simulink model "WF_offshore"  (R2024a)
settings: Solver=VariableStepAuto  StartTime=0  StopTime=1  RelTol=1e-3
values from neighbouring files (symbols this model uses):
  c_c = 0.177e-6    (= 1.77e-07)    [WF_onshore_SSO_GFL.m]    (also in WF_physical_param_offshore_supersynchronous.m = cable_220(i,6)*1e-9; WF_physical_param_onshore_SSO_020625.m = cable_220(i,6)*1e-9; initialize_params_agg.m)
  c_c_eff = c_c*n_cables    [WF_onshore_SSO_GFL.m]    (also in WF_physical_param_offshore_supersynchronous.m; WF_physical_param_onshore_SSO_020625.m; initialize_params_agg.m)
  cvtr = initialize_NR_VSC_GF(cvtr)    [NR_steadystate_VSC_GF.m]    (also in WF_onshore_SSO_GFL.m = setfield(cvtr,'parameters', p_vary.name,p_vary.val(i)); WF_physical_param_offshore_supersynchronous.m = setfield(cvtr,'parameters', p_vary.name,p_vary.val(i)); WF_physical_param_onshore_SSO_020625.m = setfield(cvtr,'parameters', p_vary.name,p_vary.val(i)); impedance_WT_blackbox.m = base_values(cvtr))
  D_C = 10:4:100    [WF_onshore_SSO_GFL.m]    (also in WF_parameter_variation.m = 10:4:150; WF_physical_param.m = 10:4:150; WF_physical_param_offshore_supersynchronous.m = 50; WF_physical_param_onshore_SSO_020625.m = 50)
  enable_pll = 1    [impedance_WT_agg.m]    (also in initialize_WT_agg.m; initialize_WT_default_gfl.m; initialize_WT_default_offshore_super.m)
  f1 = 50    [WF_onshore_SSO_GFL.m]    (also in WF_physical_param_offshore_supersynchronous.m; WF_physical_param_onshore_SSO_020625.m; initialize_params_agg.m)
  i = 1    [WF_physical_param_offshore_supersynchronous.m]    (also in WF_physical_param_onshore_SSO_020625.m)
  L = inv(R)    [participation_factors_VSC_GF.m]
  l_c = 0.386e-3    (= 0.000386)    [WF_onshore_SSO_GFL.m]    (also in WF_physical_param_offshore_supersynchronous.m = cable_220(i,5)*1e-3; WF_physical_param_onshore_SSO_020625.m = cable_220(i,5)*1e-3; initialize_params_agg.m)
  l_c_eff = l_c/n_cables    [WF_onshore_SSO_GFL.m]    (also in WF_physical_param_offshore_supersynchronous.m; WF_physical_param_onshore_SSO_020625.m; initialize_params_agg.m)
  L_comp = sqrt(2)*l_comp*(Z_b_G/(2*pi*f1))    [WF_physical_param.m]    (also in WF_physical_param_offshore_supersynchronous.m = sqrt(2)*((1/(c_c_eff/2*D_C*2*pi*f1))-(l_tf_wf*(Z_b_G)+(l_c_e; WF_physical_param_onshore_SSO_020625.m = sqrt(2)*((1/(c_c_eff/2*D_C*2*pi*f1))-(l_tf_wf*(Z_b_G)+(l_c_e; initialize_params_agg.m)
  l_OH = 0.2    [WF_onshore_SSO_GFL.m]    (also in WF_physical_param_offshore_supersynchronous.m = 0.1; WF_physical_param_onshore_SSO_020625.m = 0.1; initialize_params_agg.m = 0.1)
  l_tf_wf = tf_params(2,2)    [IM_WF_agg.m]    (also in WF_onshore_SSO_GFL.m = 0.05; WF_physical_param_offshore_supersynchronous.m = 0.05; WF_physical_param_onshore_SSO_020625.m = 0.05; initialize_params_agg.m = 0.05)
  l_tf_wt = tf_params(1,2)    [IM_WF_agg.m]    (also in WF_onshore_SSO_GFL.m = 0.0392; WF_physical_param_offshore_supersynchronous.m = 0.0392; WF_physical_param_onshore_SSO_020625.m = 0.0392; initialize_params_agg.m = 0.0392)
  Lg = p_vary(i)*((Z_b_G/(2*pi*f1)))    [WF_onshore_SSO_GFL.m]    (also in WF_physical_param_offshore_supersynchronous.m; WF_physical_param_onshore_SSO_020625.m; initialize_params_agg.m = 0.1*((Z_b_G/(2*pi*f1))))
  Lg1 = Lg    [WF_physical_param_offshore_supersynchronous.m]    (also in WF_physical_param_onshore_SSO_020625.m)
  Lg2 = Lg    [WF_physical_param_offshore_supersynchronous.m]    (also in WF_physical_param_onshore_SSO_020625.m)
  r_c = 27e-3    (= 0.027)    [WF_onshore_SSO_GFL.m]    (also in WF_physical_param_offshore_supersynchronous.m = cable_220(i,4)*1e-3; WF_physical_param_onshore_SSO_020625.m = cable_220(i,4)*1e-3; initialize_params_agg.m)
  r_c_eff = r_c/n_cables    [WF_onshore_SSO_GFL.m]    (also in WF_physical_param_offshore_supersynchronous.m; WF_physical_param_onshore_SSO_020625.m; initialize_params_agg.m)
  r_diss = .1    (= 0.1)    [WF_physical_param_offshore_supersynchronous.m]    (also in WF_physical_param_onshore_SSO_020625.m; calculate_WF.m; initialize_params_agg.m)
  r_OH = 0.02    [WF_onshore_SSO_GFL.m]    (also in WF_physical_param_offshore_supersynchronous.m = 0.01; WF_physical_param_onshore_SSO_020625.m = 0.01; initialize_params_agg.m)
  r_tf_wf = tf_params(2,1)    [IM_WF_agg.m]    (also in WF_onshore_SSO_GFL.m = 0.005; WF_physical_param_offshore_supersynchronous.m = 0.005; WF_physical_param_onshore_SSO_020625.m = 0.005; initialize_params_agg.m = 0.005)
  r_tf_wt = tf_params(1,1)    [IM_WF_agg.m]    (also in WF_onshore_SSO_GFL.m = 0.0056; WF_physical_param_offshore_supersynchronous.m = 0.0056; WF_physical_param_onshore_SSO_020625.m = 0.0056; initialize_params_agg.m = 0.0056)
  Rg = rg*Z_b_G    [WF_onshore_SSO_GFL.m]    (also in WF_physical_param_offshore_supersynchronous.m; WF_physical_param_onshore_SSO_020625.m; initialize_params_agg.m = 0.01*Z_b_G)
  Sb_WF = (3*1)*5e6    (= 15000000)    [WF_onshore_SSO_GFL.m]    (also in WF_physical_param_offshore_supersynchronous.m; WF_physical_param_onshore_SSO_020625.m; impedance_WT_blackbox.m = n_t*Sb_WT; initialize_params_agg.m = 1000000000)
  Sb_WT = 5e6    (= 5000000)    [IM_WF.m]    (also in WF_onshore_SSO_GFL.m; WF_physical_param_offshore_supersynchronous.m; WF_physical_param_onshore_SSO_020625.m; initialize_params_agg.m)
  selector_current_reference = 3    [impedance_WT_agg.m]    (also in initialize_WT_agg.m; initialize_WT_default_gfl.m; initialize_WT_default_offshore_super.m)
  selector_omega_reference = 1    [impedance_WT_agg.m]    (also in initialize_WT_agg.m; initialize_WT_default_gfl.m; initialize_WT_default_offshore_super.m)
  V_coll = 33e3    (= 33000)    [WF_onshore_SSO_GFL.m]    (also in WF_physical_param_offshore_supersynchronous.m; WF_physical_param_onshore_SSO_020625.m; initialize_params_agg.m)
  V_trans = 220e3    (= 220000)    [WF_onshore_SSO_GFL.m]    (also in WF_physical_param_offshore_supersynchronous.m; WF_physical_param_onshore_SSO_020625.m; initialize_params_agg.m)
  Z_b_G = (V_trans/sqrt(3/2))^2/Sb_WF    [WF_onshore_SSO_GFL.m]    (also in WF_physical_param_offshore_supersynchronous.m = (V_b_trans)^2/Sb_WF; WF_physical_param_onshore_SSO_020625.m = (V_b_trans)^2/Sb_WF; initialize_params_agg.m = (V_b_trans)^2/Sb_WF)
undefined symbols (not defined in the file or in its folder): opts, R
libraries: spsSeriesRLCBranchLib x105, simulink_extras x104, simulink x52, spsThreePhaseVIMeasurementLib x42, spsControlledVoltageSourceLib x42, spsGroundLib x41, spsThreePhaseTransformerTwoWindingsLib x14, powerlib_extras x13, spsVariableInductorLib x9, spsIdealSwitchLib x6, spsVariableCapacitorLib x6, spsThreePhaseSeriesRLCBranchLib x4
(part 7 of 13)

== system WF_offshore/WT_MF8/Inverse Park1 ==
  x_dq : Inport
  delta : Inport  Port=2
  Demux1 : Demux  Outputs=2
  Fcn : Fcn  Expr=cos(u(3))*u(1)-sin(u(3))*u(2)
  Fcn1 : Fcn  Expr=cos(u(3)-2/3*pi)*u(1)-sin(u(3)-2/3*pi)*u(2)
  Fcn2 : Fcn  Expr=cos(u(3)+2/3*pi)*u(1)-sin(u(3)+2/3*pi)*u(2)
  Mux : Mux  Inputs=3
  Mux1 : Mux  Inputs=3
  x_abc : Outport
  wires:
  delta/1 -> Mux/3
  x_dq/1 -> Demux1/1
  Mux1/1 -> x_abc/1
  Fcn2/1 -> Mux1/3
  Fcn1/1 -> Mux1/2
  Fcn/1 -> Mux1/1
  Demux1/1 -> Mux/1
  Demux1/2 -> Mux/2
  Mux/1 -> Fcn/1, Fcn2/1, Fcn1/1

== system WF_offshore/WT_MF8/Subsystem1 ==
  v_abc : Inport
  Controlled Voltage Source : spsControlledVoltageSourceLib/Controlled Voltage Source  Initialize=on  Source_Type=AC  Amplitude=0  Phase=0  Frequency=0  Measurements=None
  Controlled Voltage Source1 : spsControlledVoltageSourceLib/Controlled Voltage Source  Initialize=on  Source_Type=AC  Amplitude=0  Phase=0  Frequency=0  Measurements=None
  Controlled Voltage Source2 : spsControlledVoltageSourceLib/Controlled Voltage Source  Initialize=on  Source_Type=AC  Amplitude=0  Phase=0  Frequency=0  Measurements=None
  Demux : Demux  Outputs=3
  Ground : spsGroundLib/Ground  LConnTagsString=a
  va1 : PMIOPort  Side=Right
  vb1 : PMIOPort  Port=2  Side=Right
  vc1 : PMIOPort  Port=3  Side=Right
  wires:
  Demux/1 -> Controlled Voltage Source/1
  Demux/2 -> Controlled Voltage Source1/1
  Demux/3 -> Controlled Voltage Source2/1
  v_abc/1 -> Demux/1
  connections:
  va1/RConn1 -- Controlled Voltage Source/RConn1
  vb1/RConn1 -- Controlled Voltage Source1/RConn1
  vc1/RConn1 -- Controlled Voltage Source2/RConn1
  Ground/LConn1 -- Controlled Voltage Source2/LConn1 -- Controlled Voltage Source1/LConn1 -- Controlled Voltage Source/LConn1

== system WF_offshore/WT_MF8/Subsystem6 ==
  x_d+ix_q : Inport
  Complex to Real-Imag2 : ComplexToRealImag
  Mux : Mux  Inputs=2
  x_dq : Outport
  wires:
  x_d+ix_q/1 -> Complex to Real-Imag2/1
  Mux/1 -> x_dq/1
  Complex to Real-Imag2/2 -> Mux/2
  Complex to Real-Imag2/1 -> Mux/1

== system WF_offshore/WT_MF8/Transformations (pu and dq) ==
  i_abc_grid : Inport
  i_abc_filt : Inport  Port=2
  v_abc_grid : Inport  Port=3
  v_abc_filt : Inport  Port=4
  Thetavsm : Inport  Port=5
  Thetapll : Inport  Port=6
  3-phase Instantaneous Active & Reactive Power : powerlib_extras/Measurements/3-phase  Instantaneous  Active & Reactive Power
  Demux : Demux  Outputs=2
  Gain : Gain  Gain=1/cvtr.pu.Vb
  Gain1 : Gain  Gain=1/cvtr.pu.Ib
  Gain2 : Gain  Gain=1/cvtr.pu.Sb
  Gain4 : Gain  Gain=1/cvtr.pu.Ib
  Gain6 : Gain  Gain=1/cvtr.pu.Vb
  Park : Subsystem
  Park1 : Subsystem
  Park2 : Subsystem
  Park4 : Subsystem
  Subsystem2 : Subsystem
  Subsystem3 : Subsystem
  Subsystem4 : Subsystem
  Subsystem7 : Subsystem
  io : Outport
  il : Outport  Port=2
  p : Outport  Port=3
  q : Outport  Port=4
  vo_pll : Outport  Port=5
  vo : Outport  Port=6
  wires:
  v_abc_filt/1 -> Gain6/1, Gain/1
  Park2/1(x_dq) -> Subsystem3/1(x_dq)
  Park1/1(x_dq) -> Subsystem4/1(x_dq)
  Park/1(x_dq) -> Subsystem7/1(x_dq)
  Subsystem3/1(x_d+ix_q) -> vo/1
  Subsystem7/1(x_d+ix_q) -> il/1
  Subsystem4/1(x_d+ix_q) -> io/1
  3-phase Instantaneous Active & Reactive Power/1 -> Gain2/1
  v_abc_grid/1 -> 3-phase Instantaneous Active & Reactive Power/1
  Demux/2 -> q/1
  Thetavsm/1 -> Park/2(delta), Park2/2(delta), Park1/2(delta)
  Subsystem2/1(x_d+ix_q) -> vo_pll/1
  Thetapll/1 -> Park4/2(delta)
  i_abc_filt/1 -> Gain4/1
  Demux/1 -> p/1
  Park4/1(x_dq) -> Subsystem2/1(x_dq)
  Gain4/1 -> Park/1(x_abc)
  Gain/1 -> Park2/1(x_abc)
  Gain1/1 -> Park1/1(x_abc)
  Gain2/1 -> Demux/1
  i_abc_grid/1 -> Gain1/1, 3-phase Instantaneous Active & Reactive Power/2
  Gain6/1 -> Park4/1(x_abc)

== system WF_offshore/WT_MF8/filter capacitance1 ==
  Ground : spsGroundLib/Ground  LConnTagsString=a
  Series RLC Branch : spsSeriesRLCBranchLib/Series RLC Branch  LConnTagsString=__new0  RConnTagsString=__new0  BranchType=C  Resistance=R  Inductance=L  SetiL0=on  InitialCurrent=ia0  Capacitance=cvtr.parameters.Cf  Setx0=on  InitialVoltage=cvtr.ss.vo0a  Measurements=None
  Series RLC Branch1 : spsSeriesRLCBranchLib/Series RLC Branch  LConnTagsString=__new0  RConnTagsString=__new0  BranchType=C  Resistance=R  Inductance=L  SetiL0=on  InitialCurrent=ia0  Capacitance=cvtr.parameters.Cf  Setx0=on  InitialVoltage=cvtr.ss.vo0b  Measurements=None
  Series RLC Branch2 : spsSeriesRLCBranchLib/Series RLC Branch  LConnTagsString=__new0  RConnTagsString=__new0  BranchType=C  Resistance=R  Inductance=L  SetiL0=on  InitialCurrent=ia0  Capacitance=cvtr.parameters.Cf  Setx0=on  InitialVoltage=cvtr.ss.vo0c  Measurements=None
  Three-Phase V-I Measurement : spsThreePhaseVIMeasurementLib/Three-Phase V-I Measurement  VoltageMeasurement=phase-to-ground  SetLabelV=off  LabelV=Vabc  Vpu=off  VpuLL=off  CurrentMeasurement=no  SetLabelI=off  LabelI=Iabc  Ipu=off  Pbase=100e6  Vbase=500e3  OutputType=Complex  PhasorSimulation=off  PSBequivalent=0
  A : PMIOPort  Side=Left
  B : PMIOPort  Port=2  Side=Left
  C : PMIOPort  Port=3  Side=Left
  v_abc : Outport
  wires:
  Three-Phase V-I Measurement/1 -> v_abc/1
  connections:
  Series RLC Branch2/RConn1 -- Series RLC Branch1/RConn1 -- Ground/LConn1 -- Series RLC Branch/RConn1
  Three-Phase V-I Measurement/RConn3 -- Series RLC Branch2/LConn1
  Three-Phase V-I Measurement/RConn2 -- Series RLC Branch1/LConn1
  Three-Phase V-I Measurement/RConn1 -- Series RLC Branch/LConn1
  C/RConn1 -- Three-Phase V-I Measurement/LConn3
  B/RConn1 -- Three-Phase V-I Measurement/LConn2
  A/RConn1 -- Three-Phase V-I Measurement/LConn1

== system WF_offshore/WT_MF8/filter inductance1 ==
  Series RLC Branch : spsSeriesRLCBranchLib/Series RLC Branch  LConnTagsString=__new0  RConnTagsString=__new0  BranchType=RL  Resistance=cvtr.parameters.Rf  Inductance=cvtr.parameters.Lf  SetiL0=on  InitialCurrent=cvtr.ss.il0a  Capacitance=1e-6  Setx0=off  InitialVoltage=0  Measurements=None
  Series RLC Branch1 : spsSeriesRLCBranchLib/Series RLC Branch  LConnTagsString=__new0  RConnTagsString=__new0  BranchType=RL  Resistance=cvtr.parameters.Rf  Inductance=cvtr.parameters.Lf  SetiL0=on  InitialCurrent=cvtr.ss.il0b  Capacitance=1e-6  Setx0=off  InitialVoltage=0  Measurements=None
  Series RLC Branch2 : spsSeriesRLCBranchLib/Series RLC Branch  LConnTagsString=__new0  RConnTagsString=__new0  BranchType=RL  Resistance=cvtr.parameters.Rf  Inductance=cvtr.parameters.Lf  SetiL0=on  InitialCurrent=cvtr.ss.il0c  Capacitance=1e-6  Setx0=off  InitialVoltage=0  Measurements=None
  Three-Phase V-I Measurement : spsThreePhaseVIMeasurementLib/Three-Phase V-I Measurement  VoltageMeasurement=no  SetLabelV=off  LabelV=Vabc  Vpu=off  VpuLL=off  CurrentMeasurement=yes  SetLabelI=off  LabelI=Iabc  Ipu=off  Pbase=100e6  Vbase=500e3  OutputType=Complex  PhasorSimulation=off  PSBequivalent=0
  A : PMIOPort  Side=Left
  B : PMIOPort  Port=2  Side=Left
  C : PMIOPort  Port=3  Side=Left
  a : PMIOPort  Port=4  Side=Right
  b : PMIOPort  Port=5  Side=Right
  c : PMIOPort  Port=6  Side=Right
  i_abc : Outport
  wires:
  Three-Phase V-I Measurement/1 -> i_abc/1
  connections:
  Series RLC Branch/RConn1 -- Three-Phase V-I Measurement/LConn1
  Series RLC Branch1/RConn1 -- Three-Phase V-I Measurement/LConn2
  Series RLC Branch2/RConn1 -- Three-Phase V-I Measurement/LConn3
  A/RConn1 -- Series RLC Branch/LConn1
  a/RConn1 -- Three-Phase V-I Measurement/RConn1
  B/RConn1 -- Series RLC Branch1/LConn1
  b/RConn1 -- Three-Phase V-I Measurement/RConn2
  C/RConn1 -- Series RLC Branch2/LConn1
  c/RConn1 -- Three-Phase V-I Measurement/RConn3

== system WF_offshore/WT_MF9/Control System ==
  io : Inport
  il : Inport  Port=2
  p : Inport  Port=3
  q : Inport  Port=4
  vo_pll : Inport  Port=5
  vo : Inport  Port=6
  Add{1..4} (4 alike) : Sum
  Compare To Constant : simulink/Logic and Bit Operations/Compare To Constant  relop===  const=0  OutDataTypeStr=boolean
  Compare To Constant1 : simulink/Logic and Bit Operations/Compare To Constant  relop===  const=1  OutDataTypeStr=boolean
  Compare To Constant2 : simulink/Logic and Bit Operations/Compare To Constant  relop===  const=2  OutDataTypeStr=boolean
  Compare To Constant3 : simulink/Logic and Bit Operations/Compare To Constant  relop===  const=3  OutDataTypeStr=boolean
  Current controller : Subsystem
  Goto2 : Goto  Commented=on  GotoTag=d_pref  TagVisibility=global
  Goto3 : Goto  Commented=on  GotoTag=d_qref  TagVisibility=global
  Goto4 : Goto  Commented=on  GotoTag=d_Oref  TagVisibility=global
  Goto6 : Goto  Commented=on  GotoTag=d_Vref  TagVisibility=global
  Mechanical1 : Subsystem
  Memory : Memory  InitialCondition=cvtr.ss.vir0
  Multiport Switch : MultiPortSwitch  DataPortOrder=Zero-based contiguous  Inputs=4  zeroidx=on  SaturateOnIntegerOverflow=off  InputSameDT=off
  Multiport Switch1 : MultiPortSwitch  DataPortOrder=Zero-based contiguous  Inputs=2  zeroidx=on  SaturateOnIntegerOverflow=off  InputSameDT=off
  Multiport Switch2 : MultiPortSwitch  DataPortOrder=Zero-based contiguous  Inputs=2  zeroidx=on  SaturateOnIntegerOverflow=off  InputSameDT=off
  PLL1 : Subsystem
  PQ controller : Subsystem
  Step : Step  Commented=on  After=0.01  SampleTime=0
  Step1 : Step  Commented=on  Time=1.5  After=0.03  SampleTime=0
  Step2 : Step  Commented=on  Time=2  After=0.001  SampleTime=0
  Step3 : Step  Commented=on  Time=2  After=0.001  SampleTime=0
  Terminator : Terminator
  Terminator1 : Terminator
  Voltage controller DEM : Subsystem
  Voltage controller QSEM : Subsystem
  Voltage controller VCVSM : Subsystem
  delta1 : Constant  Value=cvtr.ss.pref0
  delta2 : Constant  Value=cvtr.ss.DeltaThetavsm0
  delta4 : Constant  Value=cvtr.ss.ilr0
  delta5 : Constant  Value=selector_current_reference
  delta6 : Constant  Value=selector_omega_reference
  io5 : Constant  Value=cvtr.ss.Omegavsm0
  io6 : Constant  Value=cvtr.ss.qref0
  io7 : Constant  Value=cvtr.ss.vref0
  io8 : Constant  Value=cvtr.ss.Omegaref0
  p1 : InportShadow  Port=3
  q droop1 : Subsystem
  q1 : InportShadow  Port=4
  vo3 : InportShadow  Port=6
  vo4 : InportShadow  Port=6
  vo5 : InportShadow  Port=6
  thetapll : Outport
  thetavsm : Outport  Port=2
  vir : Outport  Port=3
  wires:
  io5/1 -> Mechanical1/4(Omegavsm0)
  Voltage controller DEM/1(ilr) -> Multiport Switch/2
  Add1/1 -> [pref], Mechanical1/2(pref)
  delta4/1 -> Voltage controller DEM/4(ilr0)
  Multiport Switch/1 -> Current controller/1(ilr)
  delta2/1 -> Mechanical1/3(DeltaThetavsm0)
  Add2/1 -> [qref], q droop1/2(qref)  "qref"
  delta1/1 -> Add1/2  "pref"
  q droop1/2(qm) -> Terminator/1  "qm"
  Add4/1 -> Mechanical1/5(Omegaref)  "omegaref"
  io7/1 -> Add3/2  "vref0"
  [Omegavsm] -> Voltage controller QSEM/3(Omegavsm)
  io8/1 -> Add4/2  "omegaref0"
  Step/1 -> Add1/1, Goto2/1  "dPref"
  [ve] -> Voltage controller QSEM/1(ve)
  delta5/1 -> Compare To Constant3/1, Compare To Constant2/1, Compare To Constant1/1, Multiport Switch/1, Compare To Constant/1
  io6/1 -> Add2/2  "qref0"
  Add3/1 -> q droop1/3(vref)  "vref"
  q/1 -> q droop1/1(q)
  [Omegavsm] -> Voltage controller VCVSM/2(Omega)
  [ve] -> Voltage controller DEM/1(ve)
  [Omegapll] -> Mechanical1/6(Omegapll)
  [Omegavsm] -> Voltage controller DEM/3(Omegavsm)
  p/1 -> Mechanical1/1(p)
  Voltage controller VCVSM/1(ilr) -> Multiport Switch/4
  vo/1 -> Voltage controller QSEM/2(vo)
  vo_pll/1 -> PLL1/1(vo)
  PLL1/2(vpll) -> Terminator1/1  "vpll"
  q droop1/1(ve) -> [ve]
  Voltage controller QSEM/1(ilr) -> Multiport Switch/3
  Memory/1 -> vir/1
  Current controller/1(vir) -> Memory/1
  p1/1 -> PQ controller/2(p)
  q1/1 -> PQ controller/4(q)
  PQ controller/1(ir) -> Multiport Switch/5
  il/1 -> Current controller/2(il)
  delta6/1 -> Multiport Switch2/1, Multiport Switch1/1
  [Omegapll] -> Current controller/3(Omega)
  Mechanical1/2(Omegavsm) -> Multiport Switch1/2  "wvsm"
  [Omegapll] -> Multiport Switch1/3
  Multiport Switch2/1 -> thetavsm/1
  Mechanical1/1(Thetavsm) -> Multiport Switch2/2  "thetavsm"
  Compare To Constant/1 -> Voltage controller DEM/Enable
  Compare To Constant1/1 -> Voltage controller QSEM/Enable
  Compare To Constant2/1 -> Voltage controller VCVSM/Enable
  Compare To Constant3/1 -> PQ controller/Enable
  Multiport Switch1/1 -> [Omegavsm]
  PLL1/1(Omegapll) -> [Omegapll]
  PLL1/3(Thetapll) -> Multiport Switch2/3, thetapll/1  "thetapll"
  io/1 -> Voltage controller VCVSM/3(io)
  vo3/1 -> Current controller/4(vo)
  vo4/1 -> Voltage controller DEM/2(vo)
  vo5/1 -> Voltage controller VCVSM/1(vo)
  [ve] -> Voltage controller VCVSM/4(ve)
  [pref] -> PQ controller/1(pref)
  [qref] -> PQ controller/3(qref)
  Step1/1 -> Goto3/1, Add2/1  "dQref"
  Step2/1 -> Add4/1, Goto4/1  "dOmegaref"
  Step3/1 -> Add3/1, Goto6/1  "dVref"

== system WF_offshore/WT_MF9/Inverse Park1 ==
  x_dq : Inport
  delta : Inport  Port=2
  Demux1 : Demux  Outputs=2
  Fcn : Fcn  Expr=cos(u(3))*u(1)-sin(u(3))*u(2)
  Fcn1 : Fcn  Expr=cos(u(3)-2/3*pi)*u(1)-sin(u(3)-2/3*pi)*u(2)
  Fcn2 : Fcn  Expr=cos(u(3)+2/3*pi)*u(1)-sin(u(3)+2/3*pi)*u(2)
  Mux : Mux  Inputs=3
  Mux1 : Mux  Inputs=3
  x_abc : Outport
  wires:
  Mux/1 -> Fcn1/1, Fcn2/1, Fcn/1
  Demux1/2 -> Mux/2
  Demux1/1 -> Mux/1
  Fcn/1 -> Mux1/1
  Fcn1/1 -> Mux1/2
  Fcn2/1 -> Mux1/3
  Mux1/1 -> x_abc/1
  x_dq/1 -> Demux1/1
  delta/1 -> Mux/3

== system WF_offshore/WT_MF9/Subsystem1 ==
  v_abc : Inport
  Controlled Voltage Source : spsControlledVoltageSourceLib/Controlled Voltage Source  Initialize=on  Source_Type=AC  Amplitude=0  Phase=0  Frequency=0  Measurements=None
  Controlled Voltage Source1 : spsControlledVoltageSourceLib/Controlled Voltage Source  Initialize=on  Source_Type=AC  Amplitude=0  Phase=0  Frequency=0  Measurements=None
  Controlled Voltage Source2 : spsControlledVoltageSourceLib/Controlled Voltage Source  Initialize=on  Source_Type=AC  Amplitude=0  Phase=0  Frequency=0  Measurements=None
  Demux : Demux  Outputs=3
  Ground : spsGroundLib/Ground  LConnTagsString=a
  va1 : PMIOPort  Side=Right
  vb1 : PMIOPort  Port=2  Side=Right
  vc1 : PMIOPort  Port=3  Side=Right
  wires:
  v_abc/1 -> Demux/1
  Demux/3 -> Controlled Voltage Source2/1
  Demux/2 -> Controlled Voltage Source1/1
  Demux/1 -> Controlled Voltage Source/1
  connections:
  Controlled Voltage Source/LConn1 -- Controlled Voltage Source1/LConn1 -- Controlled Voltage Source2/LConn1 -- Ground/LConn1
  vc1/RConn1 -- Controlled Voltage Source2/RConn1
  vb1/RConn1 -- Controlled Voltage Source1/RConn1
  va1/RConn1 -- Controlled Voltage Source/RConn1

== system WF_offshore/WT_MF9/Subsystem6 ==
  x_d+ix_q : Inport
  Complex to Real-Imag2 : ComplexToRealImag
  Mux : Mux  Inputs=2
  x_dq : Outport
  wires:
  Complex to Real-Imag2/1 -> Mux/1
  Complex to Real-Imag2/2 -> Mux/2
  Mux/1 -> x_dq/1
  x_d+ix_q/1 -> Complex to Real-Imag2/1

== system WF_offshore/WT_MF9/Transformations (pu and dq) ==
  i_abc_grid : Inport
  i_abc_filt : Inport  Port=2
  v_abc_grid : Inport  Port=3
  v_abc_filt : Inport  Port=4
  Thetavsm : Inport  Port=5
  Thetapll : Inport  Port=6
  3-phase Instantaneous Active & Reactive Power : powerlib_extras/Measurements/3-phase  Instantaneous  Active & Reactive Power
  Demux : Demux  Outputs=2
  Gain : Gain  Gain=1/cvtr.pu.Vb
  Gain1 : Gain  Gain=1/cvtr.pu.Ib
  Gain2 : Gain  Gain=1/cvtr.pu.Sb
  Gain4 : Gain  Gain=1/cvtr.pu.Ib
  Gain6 : Gain  Gain=1/cvtr.pu.Vb
  Park : Subsystem
  Park1 : Subsystem
  Park2 : Subsystem
  Park4 : Subsystem
  Subsystem2 : Subsystem
  Subsystem3 : Subsystem
  Subsystem4 : Subsystem
  Subsystem7 : Subsystem
  io : Outport
  il : Outport  Port=2
  p : Outport  Port=3
  q : Outport  Port=4
  vo_pll : Outport  Port=5
  vo : Outport  Port=6
  wires:
  Gain6/1 -> Park4/1(x_abc)
  i_abc_grid/1 -> 3-phase Instantaneous Active & Reactive Power/2, Gain1/1
  Gain2/1 -> Demux/1
  Gain1/1 -> Park1/1(x_abc)
  Gain/1 -> Park2/1(x_abc)
  Gain4/1 -> Park/1(x_abc)
  Park4/1(x_dq) -> Subsystem2/1(x_dq)
  Demux/1 -> p/1
  i_abc_filt/1 -> Gain4/1
  Thetapll/1 -> Park4/2(delta)
  Subsystem2/1(x_d+ix_q) -> vo_pll/1
  Thetavsm/1 -> Park1/2(delta), Park2/2(delta), Park/2(delta)
  Demux/2 -> q/1
  v_abc_grid/1 -> 3-phase Instantaneous Active & Reactive Power/1
  3-phase Instantaneous Active & Reactive Power/1 -> Gain2/1
  Subsystem4/1(x_d+ix_q) -> io/1
  Subsystem7/1(x_d+ix_q) -> il/1
  Subsystem3/1(x_d+ix_q) -> vo/1
  Park/1(x_dq) -> Subsystem7/1(x_dq)
  Park1/1(x_dq) -> Subsystem4/1(x_dq)
  Park2/1(x_dq) -> Subsystem3/1(x_dq)
  v_abc_filt/1 -> Gain/1, Gain6/1

== system WF_offshore/WT_MF9/filter capacitance1 ==
  Ground : spsGroundLib/Ground  LConnTagsString=a
  Series RLC Branch : spsSeriesRLCBranchLib/Series RLC Branch  LConnTagsString=__new0  RConnTagsString=__new0  BranchType=C  Resistance=R  Inductance=L  SetiL0=on  InitialCurrent=ia0  Capacitance=cvtr.parameters.Cf  Setx0=on  InitialVoltage=cvtr.ss.vo0a  Measurements=None
  Series RLC Branch1 : spsSeriesRLCBranchLib/Series RLC Branch  LConnTagsString=__new0  RConnTagsString=__new0  BranchType=C  Resistance=R  Inductance=L  SetiL0=on  InitialCurrent=ia0  Capacitance=cvtr.parameters.Cf  Setx0=on  InitialVoltage=cvtr.ss.vo0b  Measurements=None
  Series RLC Branch2 : spsSeriesRLCBranchLib/Series RLC Branch  LConnTagsString=__new0  RConnTagsString=__new0  BranchType=C  Resistance=R  Inductance=L  SetiL0=on  InitialCurrent=ia0  Capacitance=cvtr.parameters.Cf  Setx0=on  InitialVoltage=cvtr.ss.vo0c  Measurements=None
  Three-Phase V-I Measurement : spsThreePhaseVIMeasurementLib/Three-Phase V-I Measurement  VoltageMeasurement=phase-to-ground  SetLabelV=off  LabelV=Vabc  Vpu=off  VpuLL=off  CurrentMeasurement=no  SetLabelI=off  LabelI=Iabc  Ipu=off  Pbase=100e6  Vbase=500e3  OutputType=Complex  PhasorSimulation=off  PSBequivalent=0
  A : PMIOPort  Side=Left
  B : PMIOPort  Port=2  Side=Left
  C : PMIOPort  Port=3  Side=Left
  v_abc : Outport
  wires:
  Three-Phase V-I Measurement/1 -> v_abc/1
  connections:
  A/RConn1 -- Three-Phase V-I Measurement/LConn1
  B/RConn1 -- Three-Phase V-I Measurement/LConn2
  C/RConn1 -- Three-Phase V-I Measurement/LConn3
  Three-Phase V-I Measurement/RConn1 -- Series RLC Branch/LConn1
  Three-Phase V-I Measurement/RConn2 -- Series RLC Branch1/LConn1
  Three-Phase V-I Measurement/RConn3 -- Series RLC Branch2/LConn1
  Series RLC Branch/RConn1 -- Ground/LConn1 -- Series RLC Branch1/RConn1 -- Series RLC Branch2/RConn1

== system WF_offshore/WT_MF9/filter inductance1 ==
  Series RLC Branch : spsSeriesRLCBranchLib/Series RLC Branch  LConnTagsString=__new0  RConnTagsString=__new0  BranchType=RL  Resistance=cvtr.parameters.Rf  Inductance=cvtr.parameters.Lf  SetiL0=on  InitialCurrent=cvtr.ss.il0a  Capacitance=1e-6  Setx0=off  InitialVoltage=0  Measurements=None
  Series RLC Branch1 : spsSeriesRLCBranchLib/Series RLC Branch  LConnTagsString=__new0  RConnTagsString=__new0  BranchType=RL  Resistance=cvtr.parameters.Rf  Inductance=cvtr.parameters.Lf  SetiL0=on  InitialCurrent=cvtr.ss.il0b  Capacitance=1e-6  Setx0=off  InitialVoltage=0  Measurements=None
  Series RLC Branch2 : spsSeriesRLCBranchLib/Series RLC Branch  LConnTagsString=__new0  RConnTagsString=__new0  BranchType=RL  Resistance=cvtr.parameters.Rf  Inductance=cvtr.parameters.Lf  SetiL0=on  InitialCurrent=cvtr.ss.il0c  Capacitance=1e-6  Setx0=off  InitialVoltage=0  Measurements=None
  Three-Phase V-I Measurement : spsThreePhaseVIMeasurementLib/Three-Phase V-I Measurement  VoltageMeasurement=no  SetLabelV=off  LabelV=Vabc  Vpu=off  VpuLL=off  CurrentMeasurement=yes  SetLabelI=off  LabelI=Iabc  Ipu=off  Pbase=100e6  Vbase=500e3  OutputType=Complex  PhasorSimulation=off  PSBequivalent=0
  A : PMIOPort  Side=Left
  B : PMIOPort  Port=2  Side=Left
  C : PMIOPort  Port=3  Side=Left
  a : PMIOPort  Port=4  Side=Right
  b : PMIOPort  Port=5  Side=Right
  c : PMIOPort  Port=6  Side=Right
  i_abc : Outport
  wires:
  Three-Phase V-I Measurement/1 -> i_abc/1
  connections:
  c/RConn1 -- Three-Phase V-I Measurement/RConn3
  C/RConn1 -- Series RLC Branch2/LConn1
  b/RConn1 -- Three-Phase V-I Measurement/RConn2
  B/RConn1 -- Series RLC Branch1/LConn1
  a/RConn1 -- Three-Phase V-I Measurement/RConn1
  A/RConn1 -- Series RLC Branch/LConn1
  Series RLC Branch2/RConn1 -- Three-Phase V-I Measurement/LConn3
  Series RLC Branch1/RConn1 -- Three-Phase V-I Measurement/LConn2
  Series RLC Branch/RConn1 -- Three-Phase V-I Measurement/LConn1

== system WF_offshore/WT_MF1/Control System/Current controller ==
  note: Active damping
  note: Feedforward
  note: Decoupling term
  note: PI regulator
  ilr : Inport
  il : Inport  Port=2
  Omega : Inport  Port=3
  vo : Inport  Port=4
  Gain : Gain  Gain=cvtr.parameters.kpc
  Gain1 : Gain
  Gain2 : Gain  Gain=cvtr.parameters.kic
  Gain3 : Gain  Gain=1i*cvtr.parameters.lf
  Gain4 : Gain  Gain=cvtr.parameters.kffv
  Gain5 : Gain  Gain=cvtr.parameters.kad
  Product : Product  RndMeth=Zero
  Subsystem : Subsystem
  Subsystem1 : Subsystem  mask{Omega=cvtr.parameters.Omegaad, xd0=cvtr.ss.Phid0, xq0=cvtr.ss.Phiq0}
  Subtract1 : Sum  Inputs=|++
  Subtract2 : Sum  Inputs=|++
  Subtract3 : Sum  Inputs=|+-
  Subtract4 : Sum  Inputs=|+-
  Subtract5 : Sum  Inputs=|++
  Subtract6 : Sum  Inputs=|+-
  delta1 : Constant  Value=cvtr.ss.Gamma0
  il1 : InportShadow  Port=2
  vo1 : InportShadow  Port=4
  vir : Outport
  wires:
  Gain2/1 -> Subtract1/2
  Gain3/1 -> Subtract2/2
  Product/1 -> Gain3/1
  Omega/1 -> Product/2
  vo/1 -> Gain4/1
  Gain4/1 -> Subtract5/2
  Gain5/1 -> Subtract6/2
  Subtract4/1 -> Gain5/1
  delta1/1 -> Subsystem/2(x0)
  il/1 -> Subtract3/2
  Subsystem/1(x/s) -> Gain2/1  "Gamma"
  il1/1 -> Product/1
  Subtract1/1 -> Subtract2/1
  vo1/1 -> Subsystem1/1(in), Subtract4/1
  Subsystem1/1(out) -> Subtract4/2
  Subtract2/1 -> Subtract5/1
  Subtract5/1 -> Subtract6/1
  Gain/1 -> Subtract1/1
  Subtract6/1 -> Gain1/1
  Gain1/1 -> vir/1
  Subtract3/1 -> Subsystem/1(x), Gain/1
  ilr/1 -> Subtract3/1

== system WF_offshore/WT_MF1/Control System/Mechanical1 ==
  p : Inport
  pref : Inport  Port=2
  DeltaThetavsm0 : Inport  Port=3
  Omegavsm0 : Inport  Port=4
  Omegaref : Inport  Port=5
  Omegapll : Inport  Port=6
  Constant : Constant  Value=enable_pll
  Gain : Gain  Gain=1/cvtr.parameters.ta
  Gain1 : Gain  Gain=cvtr.parameters.kd
  Gain2 : Gain  Gain=cvtr.parameters.kdrpOmega
  Gain3 : Gain  Gain=cvtr.pu.Omegab
  Integrator1 : Integrator  InitialConditionSource=external
  Integrator2 : Integrator  InitialConditionSource=external
  Subtract : Sum  Inputs=-+--
  Subtract1 : Sum  Inputs=-+
  Subtract2 : Sum  Inputs=-+
  Switch : Switch  Criteria=u2 > Threshold  SaturateOnIntegerOverflow=off  InputSameDT=off
  Transfer Fcn (with initial outputs) : simulink_extras/Additional Linear/Transfer Fcn (with initial outputs)  N=[cvtr.parameters.Omegadf]  D="[1  cvtr.parameters.Omegadf]"  Y0=cvtr.ss.Kappa0  U0=cvtr.ss.Kappa0
  Thetavsm : Outport
  Omegavsm : Outport  Port=2
  wires:
  DeltaThetavsm0/1 -> Integrator1/2
  p/1 -> Subtract/1
  pref/1 -> Subtract/2
  Subtract/1 -> Gain/1
  Gain1/1 -> Subtract/3
  Subtract1/1 -> Gain1/1
  Omegavsm0/1 -> Integrator2/2
  Gain/1 -> Integrator2/1
  Omegaref/1 -> Subtract2/1
  Subtract2/1 -> Gain2/1
  Gain2/1 -> Subtract/4
  Gain3/1 -> Integrator1/1
  Omegapll/1 -> Switch/1
  Constant/1 -> Switch/2
  Transfer Fcn (with initial outputs)/1 -> Switch/3
  Integrator2/1 -> Gain3/1, Transfer Fcn (with initial outputs)/1, Subtract2/2, Subtract1/2, Omegavsm/1
  Switch/1 -> Subtract1/1
  Integrator1/1 -> Thetavsm/1

== system WF_offshore/WT_MF1/Control System/PLL1 ==
  note: DeltaOmegapll
  vo : Inport
  Add : Sum
  Add3 : Sum
  Constant : Constant  Value=cvtr.ss.Epsilonpll0
  Constant1 : Constant  Value=cvtr.ss.DeltaThetapll0
  Constant3 : Constant  Value=-cvtr.ss.DeltaThetapll0
  Constant4 : Constant  Value=cvtr.parameters.Omegan
  Demux : Demux  Outputs=2
  Demux1 : Demux  Outputs=2
  Gain : Gain  Gain=cvtr.parameters.kppll
  Gain1 : Gain  Gain=cvtr.pu.Omegab
  Gain2 : Gain  Gain=cvtr.parameters.kipll
  Integrator1 : Integrator  InitialConditionSource=external
  Integrator2 : Integrator  InitialConditionSource=external
  Multiport Switch1 : MultiPortSwitch  DataPortOrder=Zero-based contiguous  Inputs=2  zeroidx=on  SaturateOnIntegerOverflow=off  InputSameDT=off
  Mux : Mux  Inputs=2
  Subsystem1 : Subsystem
  Subsystem3 : Subsystem
  Terminator : Terminator
  Terminator1 : Terminator
  Transfer Fcn (with initial outputs) : simulink_extras/Additional Linear/Transfer Fcn (with initial outputs)  N=[cvtr.parameters.Omegalppll]  D="[1  cvtr.parameters.Omegalppll]"  Y0=real(cvtr.ss.vpll0)  U0=real(cvtr.ss.vpll0)
  Transfer Fcn (with initial outputs)1 : simulink_extras/Additional Linear/Transfer Fcn (with initial outputs)  N=[cvtr.parameters.Omegalppll]  D="[1  cvtr.parameters.Omegalppll]"  Y0=imag(cvtr.ss.vpll0)  U0=imag(cvtr.ss.vpll0)
  Trigonometric Function : Trigonometry  Operator=atan2
  delta6 : Constant  Value=selector_omega_reference
  Omegapll : Outport
  vpll : Outport  Port=2
  Thetapll : Outport  Port=3
  wires:
  vo/1 -> Subsystem1/1(x_d+ix_q)
  Subsystem1/1(x_dq) -> Demux/1
  Transfer Fcn (with initial outputs)1/1 -> Trigonometric Function/1, Mux/2
  Trigonometric Function/1 -> Integrator2/1, Gain/1
  Gain/1 -> Add/1
  Constant/1 -> Integrator2/2
  Gain2/1 -> Add/2
  Add/1 -> Add3/2
  Subsystem3/1(x_d+ix_q) -> vpll/1
  Add3/1 -> Omegapll/1, Gain1/1
  Constant4/1 -> Add3/1
  Gain1/1 -> Integrator1/1
  Mux/1 -> Demux1/1, Subsystem3/1(x_dq)
  Demux1/2 -> Terminator1/1  "vpll_q"
  Demux1/1 -> Terminator/1  "vpll_d"
  Demux/1 -> Transfer Fcn (with initial outputs)/1
  Transfer Fcn (with initial outputs)/1 -> Mux/1, Trigonometric Function/2
  Integrator2/1 -> Gain2/1
  Integrator1/1 -> Thetapll/1
  Constant3/1 -> Multiport Switch1/3
  delta6/1 -> Multiport Switch1/1
  Constant1/1 -> Multiport Switch1/2
  Multiport Switch1/1 -> Integrator1/2
  Demux/2 -> Transfer Fcn (with initial outputs)1/1

== system WF_offshore/WT_MF1/Control System/PQ controller ==
  note: PI regulator
  note: PI regulator
  pref : Inport
  p : Inport  Port=2
  qref : Inport  Port=3
  q : Inport  Port=4
  Enable : EnablePort
  Gain : Gain  Gain=cvtr.parameters.kpp
  Gain1 : Gain  Gain=cvtr.parameters.kpq
  Gain2 : Gain  Gain=cvtr.parameters.kip
  Gain3 : Gain  Gain=cvtr.parameters.kiq
  Gain4 : Gain
  Gain5 : Gain  Gain=-1
  Integrator1 : Integrator  InitialConditionSource=external
  Integrator2 : Integrator  InitialConditionSource=external
  Mux : Mux  Inputs=2
  Subsystem3 : Subsystem
  Subtract1 : Sum  Inputs=|++
  Subtract2 : Sum  Inputs=|++
  Subtract3 : Sum  Inputs=|+-
  Subtract4 : Sum  Inputs=|+-
  delta1 : Constant  Value=cvtr.ss.GammaSd0
  delta2 : Constant  Value=cvtr.ss.GammaSq0
  ir : Outport
  wires:
  Gain/1 -> Subtract1/1
  Integrator1/1 -> Gain2/1
  p/1 -> Subtract3/2
  Subtract3/1 -> Integrator1/1, Gain/1
  delta1/1 -> Integrator1/2
  Gain2/1 -> Subtract1/2
  pref/1 -> Subtract3/1
  qref/1 -> Subtract4/1
  Gain3/1 -> Subtract2/2
  delta2/1 -> Integrator2/2
  Subtract4/1 -> Integrator2/1, Gain1/1
  q/1 -> Subtract4/2
  Integrator2/1 -> Gain3/1
  Gain1/1 -> Subtract2/1
  Mux/1 -> Subsystem3/1(x_dq)
  Subtract1/1 -> Gain4/1
  Subtract2/1 -> Gain5/1
  Subsystem3/1(x_d+ix_q) -> ir/1
  Gain5/1 -> Mux/2
  Gain4/1 -> Mux/1

== system WF_offshore/WT_MF1/Control System/Voltage controller DEM ==
  ve : Inport
  vo : Inport  Port=2
  Omegavsm : Inport  Port=3
  ilr0 : Inport  Port=4
  Enable : EnablePort
  Gain : Gain  Gain=cvtr.pu.Omegab/cvtr.parameters.ls
  Gain1 : Gain  Gain=cvtr.pu.Omegab/cvtr.parameters.ls
  Gain2 : Gain  Gain=cvtr.pu.Omegab*cvtr.parameters.rs/cvtr.parameters.ls
  Gain3 : Gain  Gain=1i*cvtr.pu.Omegab
  Product : Product  RndMeth=Zero
  Subsystem : Subsystem
  Subtract : Sum  Inputs=+---
  ilr : Outport
  wires:
  Omegavsm/1 -> Product/2
  Product/1 -> Gain3/1
  Gain3/1 -> Subtract/4
  Gain2/1 -> Subtract/3
  Subtract/1 -> Subsystem/1(x)
  Gain1/1 -> Subtract/2
  vo/1 -> Gain1/1
  Gain/1 -> Subtract/1
  ve/1 -> Gain/1
  Subsystem/1(x/s) -> Product/1, Gain2/1, ilr/1
  ilr0/1 -> Subsystem/2(x0)

== system WF_offshore/WT_MF1/Control System/Voltage controller QSEM ==
  ve : Inport
  vo : Inport  Port=2
  Omegavsm : Inport  Port=3
  Enable : EnablePort
  Constant : Constant  Value=cvtr.pu.Omegab*cvtr.parameters.rs/cvtr.parameters.ls
  Demux : Demux  Outputs=2
  Demux1 : Demux  Outputs=2
  Divide : Product  Inputs=*/
  Gain : Gain  Gain=cvtr.pu.Omegab/cvtr.parameters.ls
  Gain1 : Gain  Gain=cvtr.pu.Omegab/cvtr.parameters.ls
  Gain3 : Gain  Gain=1i*cvtr.pu.Omegab
  Mux : Mux  Inputs=2
  Subsystem2 : Subsystem
  Subsystem3 : Subsystem
  Subtract : Sum  Inputs=+-
  Subtract1 : Sum
  Terminator : Terminator
  Terminator1 : Terminator
  Transfer Fcn (with initial outputs) : simulink_extras/Additional Linear/Transfer Fcn (with initial outputs)  N=[cvtr.parameters.Omegavo]  D="[1  cvtr.parameters.Omegavo]"  Y0=cvtr.ss.vomd0  U0=cvtr.ss.vomd0
  Transfer Fcn (with initial outputs)1 : simulink_extras/Additional Linear/Transfer Fcn (with initial outputs)  N=[cvtr.parameters.Omegavo]  D="[1  cvtr.parameters.Omegavo]"  Y0=cvtr.ss.vomq0  U0=cvtr.ss.vomq0
  ilr : Outport
  wires:
  Omegavsm/1 -> Gain3/1
  Gain3/1 -> Subtract1/2
  Gain1/1 -> Subtract/2
  Gain/1 -> Subtract/1
  ve/1 -> Gain/1
  Subtract/1 -> Divide/1
  Constant/1 -> Subtract1/1
  Divide/1 -> ilr/1
  Subtract1/1 -> Divide/2
  vo/1 -> Subsystem2/1(x_d+ix_q)
  Subsystem2/1(x_dq) -> Demux/1
  Transfer Fcn (with initial outputs)/1 -> Mux/1
  Mux/1 -> Demux1/1, Subsystem3/1(x_dq)
  Subsystem3/1(x_d+ix_q) -> Gain1/1
  Demux1/1 -> Terminator/1  "vomd?"
  Demux1/2 -> Terminator1/1  "vomq?"
  Demux/1 -> Transfer Fcn (with initial outputs)/1
  Demux/2 -> Transfer Fcn (with initial outputs)1/1
  Transfer Fcn (with initial outputs)1/1 -> Mux/2

== system WF_offshore/WT_MF1/Control System/Voltage controller VCVSM ==
  note: Voltage controller
  note: Feedforward
  note: Decoupling term
  note: PI regulator
  vo : Inport
  Omega : Inport  Port=2
  io : Inport  Port=3
  ve : Inport  Port=4
  Enable : EnablePort
  Gain : Gain  Gain=cvtr.parameters.kpv
  Gain1 : Gain  Gain=cvtr.parameters.rs
  Gain2 : Gain  Gain=cvtr.parameters.kiv
  Gain3 : Gain  Gain=1i*cvtr.parameters.cf
  Gain4 : Gain  Gain=cvtr.parameters.kffi
  Gain5 : Gain  Gain=1i*cvtr.parameters.ls
  Omega1 : InportShadow  Port=2
  Product : Product  RndMeth=Zero
  Product1 : Product
  Subsystem : Subsystem
  Subtract : Sum  Inputs=+--
  Subtract1 : Sum  Inputs=|++
  Subtract2 : Sum  Inputs=|++
  Subtract3 : Sum  Inputs=|+-
  Subtract5 : Sum  Inputs=|++
  delta1 : Constant  Value=cvtr.ss.Xi0
  io1 : InportShadow  Port=3
  vo1 : InportShadow
  ilr : Outport
  wires:
  Subtract/1 -> Subtract3/1  "vor"
  Gain/1 -> Subtract1/1
  Gain2/1 -> Subtract1/2
  Gain3/1 -> Subtract2/2
  Product/1 -> Gain3/1
  Omega/1 -> Product/2
  io/1 -> Gain4/1
  Gain4/1 -> Subtract5/2
  delta1/1 -> Subsystem/2(x0)
  Subtract3/1 -> Gain/1, Subsystem/1(x)
  vo/1 -> Subtract3/2
  Subsystem/1(x/s) -> Gain2/1  "Xi"
  vo1/1 -> Product/1
  Subtract1/1 -> Subtract2/1
  Subtract2/1 -> Subtract5/1
  Subtract5/1 -> ilr/1
  io1/1 -> Gain1/1, Product1/1
  Omega1/1 -> Product1/2
  Gain5/1 -> Subtract/3
  Product1/1 -> Gain5/1
  ve/1 -> Subtract/1
  Gain1/1 -> Subtract/2

== system WF_offshore/WT_MF1/Control System/q droop1 ==
  q : Inport
  qref : Inport  Port=2
  vref : Inport  Port=3
  Gain3 : Gain  Gain=cvtr.parameters.kdrpq
  Subtract : Sum
  Subtract3 : Sum  Inputs=-+
  Transfer Fcn (with initial outputs) : simulink_extras/Additional Linear/Transfer Fcn (with initial outputs)  N=[cvtr.parameters.Omegaqf]  D="[1  cvtr.parameters.Omegaqf]"  Y0=cvtr.ss.q0  U0=cvtr.ss.q0
  ve : Outport
  qm : Outport  Port=2
  wires:
  vref/1 -> Subtract/2
  qref/1 -> Subtract3/2
  Transfer Fcn (with initial outputs)/1 -> Subtract3/1, qm/1
  Subtract3/1 -> Gain3/1
  Gain3/1 -> Subtract/1
  Subtract/1 -> ve/1
  q/1 -> Transfer Fcn (with initial outputs)/1

== system WF_offshore/WT_MF1/Transformations (pu and dq)/Park ==
  x_abc : Inport
  delta : Inport  Port=2
  Demux1 : Demux  Outputs=3
  Fcn : Fcn  Expr=2/3*(cos(u(4))*u(1)+cos(u(4)-2/3*pi)*u(2)+cos(u(4)+2/3*pi)*u(3))
  Fcn1 : Fcn  Expr=-2/3*(sin(u(4))*u(1)+sin(u(4)-2/3*pi)*u(2)+sin(u(4)+2/3*pi)*u(3))
  Mux : Mux
  Mux1 : Mux  Inputs=2
  x_dq : Outport
  wires:
  Demux1/1 -> Mux/1
  Demux1/2 -> Mux/2
  Demux1/3 -> Mux/3
  x_abc/1 -> Demux1/1
  delta/1 -> Mux/4
  Mux/1 -> Fcn/1, Fcn1/1
  Fcn/1 -> Mux1/1
  Fcn1/1 -> Mux1/2
  Mux1/1 -> x_dq/1

== system WF_offshore/WT_MF1/Transformations (pu and dq)/Park1 ==
  x_abc : Inport
  delta : Inport  Port=2
  Demux1 : Demux  Outputs=3
  Fcn : Fcn  Expr=2/3*(cos(u(4))*u(1)+cos(u(4)-2/3*pi)*u(2)+cos(u(4)+2/3*pi)*u(3))
  Fcn1 : Fcn  Expr=-2/3*(sin(u(4))*u(1)+sin(u(4)-2/3*pi)*u(2)+sin(u(4)+2/3*pi)*u(3))
  Mux : Mux
  Mux1 : Mux  Inputs=2
  x_dq : Outport
  wires:
  Mux1/1 -> x_dq/1
  Fcn1/1 -> Mux1/2
  Fcn/1 -> Mux1/1
  Mux/1 -> Fcn1/1, Fcn/1
  delta/1 -> Mux/4
  x_abc/1 -> Demux1/1
  Demux1/3 -> Mux/3
  Demux1/2 -> Mux/2
  Demux1/1 -> Mux/1

== system WF_offshore/WT_MF1/Transformations (pu and dq)/Park2 ==
  x_abc : Inport
  delta : Inport  Port=2
  Demux1 : Demux  Outputs=3
  Fcn : Fcn  Expr=2/3*(cos(u(4))*u(1)+cos(u(4)-2/3*pi)*u(2)+cos(u(4)+2/3*pi)*u(3))
  Fcn1 : Fcn  Expr=-2/3*(sin(u(4))*u(1)+sin(u(4)-2/3*pi)*u(2)+sin(u(4)+2/3*pi)*u(3))
  Mux : Mux
  Mux1 : Mux  Inputs=2
  x_dq : Outport
  wires:
  Mux1/1 -> x_dq/1
  Fcn1/1 -> Mux1/2
  Fcn/1 -> Mux1/1
  Mux/1 -> Fcn1/1, Fcn/1
  delta/1 -> Mux/4
  x_abc/1 -> Demux1/1
  Demux1/3 -> Mux/3
  Demux1/2 -> Mux/2
  Demux1/1 -> Mux/1

== system WF_offshore/WT_MF1/Transformations (pu and dq)/Park4 ==
  x_abc : Inport
  delta : Inport  Port=2
  Demux1 : Demux  Outputs=3
  Fcn : Fcn  Expr=2/3*(cos(u(4))*u(1)+cos(u(4)-2/3*pi)*u(2)+cos(u(4)+2/3*pi)*u(3))
  Fcn1 : Fcn  Expr=-2/3*(sin(u(4))*u(1)+sin(u(4)-2/3*pi)*u(2)+sin(u(4)+2/3*pi)*u(3))
  Mux : Mux
  Mux1 : Mux  Inputs=2
  x_dq : Outport
  wires:
  Mux1/1 -> x_dq/1
  Fcn1/1 -> Mux1/2
  Fcn/1 -> Mux1/1
  Mux/1 -> Fcn1/1, Fcn/1
  delta/1 -> Mux/4
  x_abc/1 -> Demux1/1
  Demux1/3 -> Mux/3
  Demux1/2 -> Mux/2
  Demux1/1 -> Mux/1

== system WF_offshore/WT_MF1/Transformations (pu and dq)/Subsystem2 ==
  x_dq : Inport
  Demux : Demux  Outputs=2
  Real-Imag to Complex : RealImagToComplex
  x_d+ix_q : Outport
  wires:
  Demux/1 -> Real-Imag to Complex/1
  Demux/2 -> Real-Imag to Complex/2
  x_dq/1 -> Demux/1
  Real-Imag to Complex/1 -> x_d+ix_q/1

== system WF_offshore/WT_MF1/Transformations (pu and dq)/Subsystem3 ==
  x_dq : Inport
  Demux : Demux  Outputs=2
  Real-Imag to Complex : RealImagToComplex
  x_d+ix_q : Outport
  wires:
  Demux/1 -> Real-Imag to Complex/1
  Demux/2 -> Real-Imag to Complex/2
  x_dq/1 -> Demux/1
  Real-Imag to Complex/1 -> x_d+ix_q/1

== system WF_offshore/WT_MF1/Transformations (pu and dq)/Subsystem4 ==
  x_dq : Inport
  Demux : Demux  Outputs=2
  Real-Imag to Complex : RealImagToComplex
  x_d+ix_q : Outport
  wires:
  Demux/1 -> Real-Imag to Complex/1
  Demux/2 -> Real-Imag to Complex/2
  x_dq/1 -> Demux/1
  Real-Imag to Complex/1 -> x_d+ix_q/1

== system WF_offshore/WT_MF1/Transformations (pu and dq)/Subsystem7 ==
  x_dq : Inport
  Demux : Demux  Outputs=2
  Real-Imag to Complex : RealImagToComplex
  x_d+ix_q : Outport
  wires:
  Real-Imag to Complex/1 -> x_d+ix_q/1
  x_dq/1 -> Demux/1
  Demux/2 -> Real-Imag to Complex/2
  Demux/1 -> Real-Imag to Complex/1

== system WF_offshore/WT_MF10/Control System/Current controller ==
  note: PI regulator
  note: Decoupling term
  note: Feedforward
  note: Active damping
  ilr : Inport
  il : Inport  Port=2
  Omega : Inport  Port=3
  vo : Inport  Port=4
  Gain : Gain  Gain=cvtr.parameters.kpc
  Gain1 : Gain
  Gain2 : Gain  Gain=cvtr.parameters.kic
  Gain3 : Gain  Gain=1i*cvtr.parameters.lf
  Gain4 : Gain  Gain=cvtr.parameters.kffv
  Gain5 : Gain  Gain=cvtr.parameters.kad
  Product : Product  RndMeth=Zero
  Subsystem : Subsystem
  Subsystem1 : Subsystem  mask{Omega=cvtr.parameters.Omegaad, xd0=cvtr.ss.Phid0, xq0=cvtr.ss.Phiq0}
  Subtract1 : Sum  Inputs=|++
  Subtract2 : Sum  Inputs=|++
  Subtract3 : Sum  Inputs=|+-
  Subtract4 : Sum  Inputs=|+-
  Subtract5 : Sum  Inputs=|++
  Subtract6 : Sum  Inputs=|+-
  delta1 : Constant  Value=cvtr.ss.Gamma0
  il1 : InportShadow  Port=2
  vo1 : InportShadow  Port=4
  vir : Outport
  wires:
  ilr/1 -> Subtract3/1
  Subtract3/1 -> Gain/1, Subsystem/1(x)
  Gain1/1 -> vir/1
  Subtract6/1 -> Gain1/1
  Gain/1 -> Subtract1/1
  Subtract5/1 -> Subtract6/1
  Subtract2/1 -> Subtract5/1
  Subsystem1/1(out) -> Subtract4/2
  vo1/1 -> Subtract4/1, Subsystem1/1(in)
  Subtract1/1 -> Subtract2/1
  il1/1 -> Product/1
  Subsystem/1(x/s) -> Gain2/1  "Gamma"
  il/1 -> Subtract3/2
  delta1/1 -> Subsystem/2(x0)
  Subtract4/1 -> Gain5/1
  Gain5/1 -> Subtract6/2
  Gain4/1 -> Subtract5/2
  vo/1 -> Gain4/1
  Omega/1 -> Product/2
  Product/1 -> Gain3/1
  Gain3/1 -> Subtract2/2
  Gain2/1 -> Subtract1/2

== system WF_offshore/WT_MF10/Control System/Mechanical1 ==
  p : Inport
  pref : Inport  Port=2
  DeltaThetavsm0 : Inport  Port=3
  Omegavsm0 : Inport  Port=4
  Omegaref : Inport  Port=5
  Omegapll : Inport  Port=6
  Constant : Constant  Value=enable_pll
  Gain : Gain  Gain=1/cvtr.parameters.ta
  Gain1 : Gain  Gain=cvtr.parameters.kd
  Gain2 : Gain  Gain=cvtr.parameters.kdrpOmega
  Gain3 : Gain  Gain=cvtr.pu.Omegab
  Integrator1 : Integrator  InitialConditionSource=external
  Integrator2 : Integrator  InitialConditionSource=external
  Subtract : Sum  Inputs=-+--
  Subtract1 : Sum  Inputs=-+
  Subtract2 : Sum  Inputs=-+
  Switch : Switch  Criteria=u2 > Threshold  SaturateOnIntegerOverflow=off  InputSameDT=off
  Transfer Fcn (with initial outputs) : simulink_extras/Additional Linear/Transfer Fcn (with initial outputs)  N=[cvtr.parameters.Omegadf]  D="[1  cvtr.parameters.Omegadf]"  Y0=cvtr.ss.Kappa0  U0=cvtr.ss.Kappa0
  Thetavsm : Outport
  Omegavsm : Outport  Port=2
  wires:
  Integrator1/1 -> Thetavsm/1
  Switch/1 -> Subtract1/1
  Integrator2/1 -> Omegavsm/1, Subtract1/2, Subtract2/2, Transfer Fcn (with initial outputs)/1, Gain3/1
  Transfer Fcn (with initial outputs)/1 -> Switch/3
  Constant/1 -> Switch/2
  Omegapll/1 -> Switch/1
  Gain3/1 -> Integrator1/1
  Gain2/1 -> Subtract/4
  Subtract2/1 -> Gain2/1
  Omegaref/1 -> Subtract2/1
  Gain/1 -> Integrator2/1
  Omegavsm0/1 -> Integrator2/2
  Subtract1/1 -> Gain1/1
  Gain1/1 -> Subtract/3
  Subtract/1 -> Gain/1
  pref/1 -> Subtract/2
  p/1 -> Subtract/1
  DeltaThetavsm0/1 -> Integrator1/2

== system WF_offshore/WT_MF10/Control System/PLL1 ==
  note: DeltaOmegapll
  vo : Inport
  Add : Sum
  Add3 : Sum
  Constant : Constant  Value=cvtr.ss.Epsilonpll0
  Constant1 : Constant  Value=cvtr.ss.DeltaThetapll0
  Constant3 : Constant  Value=-cvtr.ss.DeltaThetapll0
  Constant4 : Constant  Value=cvtr.parameters.Omegan
  Demux : Demux  Outputs=2
  Demux1 : Demux  Outputs=2
  Gain : Gain  Gain=cvtr.parameters.kppll
  Gain1 : Gain  Gain=cvtr.pu.Omegab
  Gain2 : Gain  Gain=cvtr.parameters.kipll
  Integrator1 : Integrator  InitialConditionSource=external
  Integrator2 : Integrator  InitialConditionSource=external
  Multiport Switch1 : MultiPortSwitch  DataPortOrder=Zero-based contiguous  Inputs=2  zeroidx=on  SaturateOnIntegerOverflow=off  InputSameDT=off
  Mux : Mux  Inputs=2
  Subsystem1 : Subsystem
  Subsystem3 : Subsystem
  Terminator : Terminator
  Terminator1 : Terminator
  Transfer Fcn (with initial outputs) : simulink_extras/Additional Linear/Transfer Fcn (with initial outputs)  N=[cvtr.parameters.Omegalppll]  D="[1  cvtr.parameters.Omegalppll]"  Y0=real(cvtr.ss.vpll0)  U0=real(cvtr.ss.vpll0)
  Transfer Fcn (with initial outputs)1 : simulink_extras/Additional Linear/Transfer Fcn (with initial outputs)  N=[cvtr.parameters.Omegalppll]  D="[1  cvtr.parameters.Omegalppll]"  Y0=imag(cvtr.ss.vpll0)  U0=imag(cvtr.ss.vpll0)
  Trigonometric Function : Trigonometry  Operator=atan2
  delta6 : Constant  Value=selector_omega_reference
  Omegapll : Outport
  vpll : Outport  Port=2
  Thetapll : Outport  Port=3
  wires:
  Demux/2 -> Transfer Fcn (with initial outputs)1/1
  Multiport Switch1/1 -> Integrator1/2
  Constant1/1 -> Multiport Switch1/2
  delta6/1 -> Multiport Switch1/1
  Constant3/1 -> Multiport Switch1/3
  Integrator1/1 -> Thetapll/1
  Integrator2/1 -> Gain2/1
  Transfer Fcn (with initial outputs)/1 -> Trigonometric Function/2, Mux/1
  Demux/1 -> Transfer Fcn (with initial outputs)/1
  Demux1/1 -> Terminator/1  "vpll_d"
  Demux1/2 -> Terminator1/1  "vpll_q"
  Mux/1 -> Subsystem3/1(x_dq), Demux1/1
  Gain1/1 -> Integrator1/1
  Constant4/1 -> Add3/1
  Add3/1 -> Gain1/1, Omegapll/1
  Subsystem3/1(x_d+ix_q) -> vpll/1
  Add/1 -> Add3/2
  Gain2/1 -> Add/2
  Constant/1 -> Integrator2/2
  Gain/1 -> Add/1
  Trigonometric Function/1 -> Gain/1, Integrator2/1
  Transfer Fcn (with initial outputs)1/1 -> Mux/2, Trigonometric Function/1
  Subsystem1/1(x_dq) -> Demux/1
  vo/1 -> Subsystem1/1(x_d+ix_q)

== system WF_offshore/WT_MF10/Control System/PQ controller ==
  note: PI regulator
  note: PI regulator
  pref : Inport
  p : Inport  Port=2
  qref : Inport  Port=3
  q : Inport  Port=4
  Enable : EnablePort
  Gain : Gain  Gain=cvtr.parameters.kpp
  Gain1 : Gain  Gain=cvtr.parameters.kpq
  Gain2 : Gain  Gain=cvtr.parameters.kip
  Gain3 : Gain  Gain=cvtr.parameters.kiq
  Gain4 : Gain
  Gain5 : Gain  Gain=-1
  Integrator1 : Integrator  InitialConditionSource=external
  Integrator2 : Integrator  InitialConditionSource=external
  Mux : Mux  Inputs=2
  Subsystem3 : Subsystem
  Subtract1 : Sum  Inputs=|++
  Subtract2 : Sum  Inputs=|++
  Subtract3 : Sum  Inputs=|+-
  Subtract4 : Sum  Inputs=|+-
  delta1 : Constant  Value=cvtr.ss.GammaSd0
  delta2 : Constant  Value=cvtr.ss.GammaSq0
  ir : Outport
  wires:
  Gain4/1 -> Mux/1
  Gain5/1 -> Mux/2
  Subsystem3/1(x_d+ix_q) -> ir/1
  Subtract2/1 -> Gain5/1
  Subtract1/1 -> Gain4/1
  Mux/1 -> Subsystem3/1(x_dq)
  Gain1/1 -> Subtract2/1
  Integrator2/1 -> Gain3/1
  q/1 -> Subtract4/2
  Subtract4/1 -> Gain1/1, Integrator2/1
  delta2/1 -> Integrator2/2
  Gain3/1 -> Subtract2/2
  qref/1 -> Subtract4/1
  pref/1 -> Subtract3/1
  Gain2/1 -> Subtract1/2
  delta1/1 -> Integrator1/2
  Subtract3/1 -> Gain/1, Integrator1/1
  p/1 -> Subtract3/2
  Integrator1/1 -> Gain2/1
  Gain/1 -> Subtract1/1

== system WF_offshore/WT_MF10/Control System/Voltage controller DEM ==
  ve : Inport
  vo : Inport  Port=2
  Omegavsm : Inport  Port=3
  ilr0 : Inport  Port=4
  Enable : EnablePort
  Gain : Gain  Gain=cvtr.pu.Omegab/cvtr.parameters.ls
  Gain1 : Gain  Gain=cvtr.pu.Omegab/cvtr.parameters.ls
  Gain2 : Gain  Gain=cvtr.pu.Omegab*cvtr.parameters.rs/cvtr.parameters.ls
  Gain3 : Gain  Gain=1i*cvtr.pu.Omegab
  Product : Product  RndMeth=Zero
  Subsystem : Subsystem
  Subtract : Sum  Inputs=+---
  ilr : Outport
  wires:
  ilr0/1 -> Subsystem/2(x0)
  Subsystem/1(x/s) -> ilr/1, Gain2/1, Product/1
  ve/1 -> Gain/1
  Gain/1 -> Subtract/1
  vo/1 -> Gain1/1
  Gain1/1 -> Subtract/2
  Subtract/1 -> Subsystem/1(x)
  Gain2/1 -> Subtract/3
  Gain3/1 -> Subtract/4
  Product/1 -> Gain3/1
  Omegavsm/1 -> Product/2
